simulink model "showKeyPoint"  (R2015a)
settings: Solver=ode45  StartTime=0.0  StopTime=10.0  RelTol=1e-3
InitFcn:
  | %% DSPBuilder Start
  | alt_dspbuilder_update_model(bdroot)
  | %% DSPBuilder End
libraries: allblocks_alteradspbuilder2 x340
(part 1 of 5)
settings Model: Creator=ASUS  LastModifiedBy=ASUS

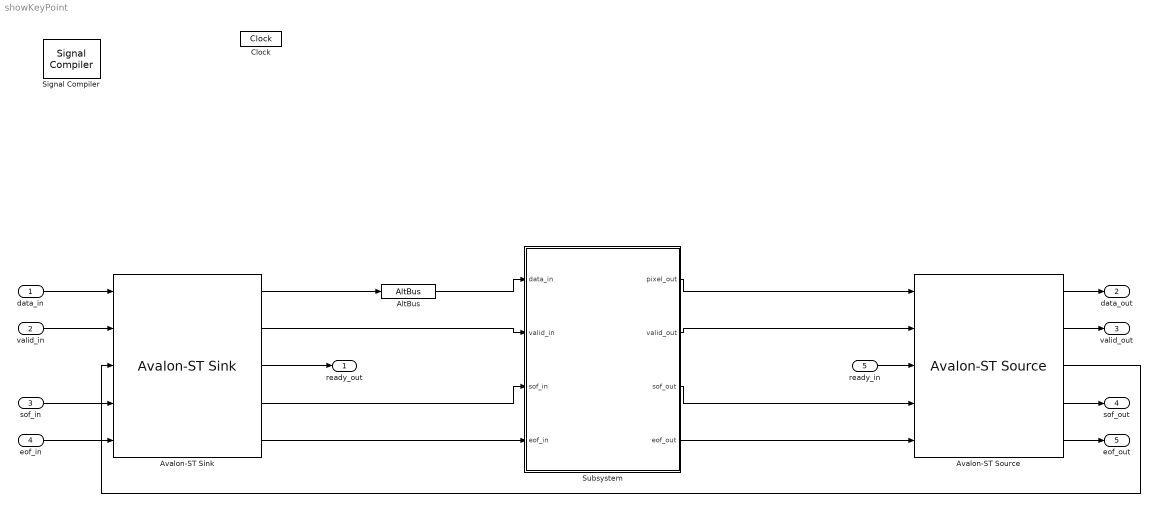
== system showKeyPoint ==
  data_in : Inport
  valid_in : Inport  Port=2
  sof_in : Inport  Port=3
  eof_in : Inport  Port=4
  ready_in : Inport  Port=5
  AltBus : allblocks_alteradspbuilder2/AltBus  BusType=Unsigned Integer  bwl=8  bwr=0  saturate=off  floatingPointInput=on  floatingPointOutput=on  logOutputs=off  logFile=C:\Users\ASUS\Desktop\sift_fpga_final\Gaussian filter 5x5\tb_gauss\gauss_AltBus.fixedpointlog
  Avalon-ST Sink : allblocks_alteradspbuilder2/Avalon-ST Sink  iofile=C:\Users\ASUS\Desktop\sift_fpga_final\Gaussian filter 5x5\tb_gauss\gauss_Avalon-ST+Sink_data.salt,C:\Users\ASUS\Desktop\sift_fpga_final\Gaussian filter 5x5\tb_gauss\gauss_Avalon-ST+Sink_valid.salt,C:\Users\ASUS\Desktop\sift_fpga_final\Gaussian filter 5x5\tb_gauss\gauss_Avalon-ST+Sink_ready.capture,C:\Users\ASUS\Desktop\sift_fpga_final\Gaussian filter 5x5\tb_gauss\gauss_Avalon-ST+Sink_startofpacket.salt,C:\Users\ASUS\Desktop\sift_fpga_final\Gaussian filter 5x5\tb_gauss\gauss_Avalon-ST+Sink_endofpacket.salt,  SpecifyClock=off  BusType=Unsigned Integer  bwl=24  bwr=0  symbolWidth=8  symbolsPerBeat=3  numOfChannels=0  numOfErrorDescriptors=0  endOfPacket=on  startOfPacket=on  empty=off  readyLatency=1  externalType=Inferred  PORTTYPE=Output
  Avalon-ST Source : allblocks_alteradspbuilder2/Avalon-ST Source  iofile=C:\Users\ASUS\Desktop\sift_fpga_final\Gaussian filter 5x5\tb_gauss\gauss_Avalon-ST+Source_data.capture,C:\Users\ASUS\Desktop\sift_fpga_final\Gaussian filter 5x5\tb_gauss\gauss_Avalon-ST+Source_valid.capture,C:\Users\ASUS\Desktop\sift_fpga_final\Gaussian filter 5x5\tb_gauss\gauss_Avalon-ST+Source_ready.salt,C:\Users\ASUS\Desktop\sift_fpga_final\Gaussian filter 5x5\tb_gauss\gauss_Avalon-ST+Source_startofpacket.capture,C:\Users\ASUS\Desktop\sift_fpga_final\Gaussian filter 5x5\tb_gauss\gauss_Avalon-ST+Source_endofpacket.capture,  SpecifyClock=off  BusType=Unsigned Integer  bwl=24  bwr=0  symbolWidth=8  symbolsPerBeat=3  numOfChannels=0  numOfErrorDescriptors=0  endOfPacket=on  startOfPacket=on  empty=off  readyLatency=1  externalType=Inferred  PORTTYPE=Input
  Clock : allblocks_alteradspbuilder2/Clock  ClockPeriod=20  ClockPeriodUnit=ns  SampleTime=1  ResetLatency=0  ResetRegisterCascadeDepth=0  SimulationStartCycle=5  PhaseOffset=0  Reset=aclr  ResetType=Active Low  Export=off
  Signal Compiler : allblocks_alteradspbuilder2/Signal Compiler  DeviceFamily=Stratix IV  DeviceName=AUTO  DisableEarlyHDLGeneration=off  EnableSignalTap=off  SignalTapDepth=128  UseBoardBlock=off  StpUseDefaultClock=on  StpClock=clock  ExportDir=.  MAX10_ProgrammingMode=Internal Flash (SDM) Single Boot
  Subsystem : Subsystem
  ready_out : Outport
  data_out : Outport  Port=2
  valid_out : Outport  Port=3
  sof_out : Outport  Port=4
  eof_out : Outport  Port=5
  wires:
  data_in/1 -> Avalon-ST Sink/1
  valid_in/1 -> Avalon-ST Sink/2
  sof_in/1 -> Avalon-ST Sink/4
  eof_in/1 -> Avalon-ST Sink/5
  ready_in/1 -> Avalon-ST Source/3
  Avalon-ST Sink/3 -> ready_out/1
  Avalon-ST Source/1 -> data_out/1
  Avalon-ST Source/2 -> valid_out/1
  Avalon-ST Source/4 -> sof_out/1
  Avalon-ST Source/5 -> eof_out/1
  Avalon-ST Sink/1 -> AltBus/1
  Subsystem/1(pixel_out) -> Avalon-ST Source/1
  Avalon-ST Sink/2 -> Subsystem/2(valid_in)
  Subsystem/2(valid_out) -> Avalon-ST Source/2
  Avalon-ST Sink/4 -> Subsystem/3(sof_in)
  Avalon-ST Sink/5 -> Subsystem/4(eof_in)
  Subsystem/3(sof_out) -> Avalon-ST Source/4
  Subsystem/4(eof_out) -> Avalon-ST Source/5
  Avalon-ST Source/3 -> Avalon-ST Sink/3
  AltBus/1 -> Subsystem/1(data_in)

== system showKeyPoint/Subsystem ==
  data_in : Inport
  valid_in : Inport  Port=2
  sof_in : Inport  Port=3
  eof_in : Inport  Port=4
  Bus Concatenation : allblocks_alteradspbuilder2/Bus Concatenation  isSigned=off  awidth=8  bwidth=8  pipeline_display=0
  Bus Concatenation1 : allblocks_alteradspbuilder2/Bus Concatenation  isSigned=off  awidth=8  bwidth=16  pipeline_display=0
  Memory Delay : allblocks_alteradspbuilder2/Memory Delay  BusType=Inferred  bwl=8  bwr=0  pipeline=4*640+28  pipeline_display=2588  ram_type=AUTO  use_ena=on  use_sclr=on  allowFloatingPointOverride=on  logOutputs=off  logFile=C:\Users\ASUS\Desktop\sift_fpga_final\Gaussian filter 5x5\tb_gauss\gauss_Subsystem_Memory+Delay.fixedpointlog
  Memory Delay1 : allblocks_alteradspbuilder2/Memory Delay  BusType=Inferred  bwl=8  bwr=0  pipeline=640*2+25  pipeline_display=1305  ram_type=AUTO  use_ena=on  use_sclr=on  allowFloatingPointOverride=on  logOutputs=off  logFile=C:\Users\ASUS\Desktop\sift_fpga_final\Gaussian filter 5x5\tb_gauss\gauss_Subsystem_Memory+Delay1.fixedpointlog
  Memory Delay2 : allblocks_alteradspbuilder2/Memory Delay  BusType=Inferred  bwl=8  bwr=0  pipeline=4*640+28  pipeline_display=2588  ram_type=AUTO  use_ena=on  use_sclr=on  allowFloatingPointOverride=on  logOutputs=off  logFile=C:\Users\ASUS\Desktop\sift_fpga_final\Gaussian filter 5x5\tb_gauss\gauss_Subsystem_Memory+Delay2.fixedpointlog
  find_keyPoint : Subsystem
  line_buff_3x3 : Subsystem
  pixel_out : Outport
  valid_out : Outport  Port=2
  sof_out : Outport  Port=3
  eof_out : Outport  Port=4
  wires:
  data_in/1 -> find_keyPoint/1(data_in), Memory Delay1/1
  Bus Concatenation/1 -> Bus Concatenation1/2
  find_keyPoint/1(is_keypoint) -> line_buff_3x3/2(is_keypoint)
  sof_in/1 -> Memory Delay/1, Memory Delay2/3, Memory Delay/3, line_buff_3x3/4(sclr), find_keyPoint/5(sclr), Memory Delay1/3, find_keyPoint/3(sof_in)
  valid_in/1 -> line_buff_3x3/3(clken), valid_out/1, Memory Delay/2, Memory Delay2/2, find_keyPoint/2(valid_in), Memory Delay1/2
  Memory Delay1/1 -> Bus Concatenation/1, Bus Concatenation1/1, Bus Concatenation/2
  line_buff_3x3/1(Out00) -> pixel_out/1
  Memory Delay/1 -> sof_out/1
  Bus Concatenation1/1 -> line_buff_3x3/1(dataIn)
  Memory Delay2/1 -> eof_out/1
  eof_in/1 -> Memory Delay2/1, find_keyPoint/4(eof_in)

== system showKeyPoint/Subsystem/find_keyPoint ==
  data_in : Inport
  valid_in : Inport  Port=2
  sof_in : Inport  Port=3
  eof_in : Inport  Port=4
  sclr : Inport  Port=5
  calculate_key_point : Subsystem
  dog_space : Subsystem
  scale_space : Subsystem
  is_keypoint : Outport
  wires:
  scale_space/3(scale2) -> dog_space/3(scale2_in)
  scale_space/1(scale4) -> dog_space/1(scale4_in)
  scale_space/2(scale3) -> dog_space/2(scale3_in)
  scale_space/4(scale1) -> dog_space/4(scale1_in)
  [pixel_in] -> scale_space/1(data_in)
  [valid_in] -> calculate_key_point/4(valid_in)
  dog_space/2(dog2_out) -> calculate_key_point/2(pixel_dog2_in)
  dog_space/1(dog3_out) -> calculate_key_point/1(pixel_dog3_in)
  valid_in/1 -> [valid_in]
  dog_space/3(dog1_out) -> calculate_key_point/3(pixel_dog1_in)
  data_in/1 -> [pixel_in]
  [valid_in] -> scale_space/2(valid_in)
  eof_in/1 -> [eof_in]
  sof_in/1 -> [sof_in]
  [valid_in] -> dog_space/5(valid_in)
  [sclr] -> dog_space/6(sclr)
  [sclr] -> calculate_key_point/5(sclr)
  [sclr] -> scale_space/3(sclr)
  calculate_key_point/1(is_KeyPoint) -> is_keypoint/1
  sclr/1 -> [sclr]

== system showKeyPoint/Subsystem/line_buff_3x3 ==
  dataIn : Inport
  is_keypoint : Inport  Port=2
  clken : Inport  Port=3
  sclr : Inport  Port=4
  Constant : allblocks_alteradspbuilder2/Constant  mask_cst=16711680  BusType=Unsigned Integer  bwl=24  bwr=0  roundMode=Truncate  satMode=Wrap  SpecifyClock=off  allowFloatingPointOverride=on  logOutputs=off  logFile=C:\Users\ASUS\Desktop\sift_fpga_final\Gaussian filter 5x5\tb_gauss\gauss_Subsystem_line%5Fbuff%5F3x3_Constant.fixedpointlog
  Constant1 : allblocks_alteradspbuilder2/Constant  mask_cst=16711680  BusType=Unsigned Integer  bwl=24  bwr=0  roundMode=Truncate  satMode=Wrap  SpecifyClock=off  allowFloatingPointOverride=on  logOutputs=off  logFile=C:\Users\ASUS\Desktop\sift_fpga_final\Gaussian filter 5x5\tb_gauss\gauss_Subsystem_line%5Fbuff%5F3x3_Constant1.fixedpointlog
  Constant2 : allblocks_alteradspbuilder2/Constant  mask_cst=16711680  BusType=Unsigned Integer  bwl=24  bwr=0  roundMode=Truncate  satMode=Wrap  SpecifyClock=off  allowFloatingPointOverride=on  logOutputs=off  logFile=C:\Users\ASUS\Desktop\sift_fpga_final\Gaussian filter 5x5\tb_gauss\gauss_Subsystem_line%5Fbuff%5F3x3_Constant2.fixedpointlog
  Constant3 : allblocks_alteradspbuilder2/Constant  mask_cst=16711680  BusType=Unsigned Integer  bwl=24  bwr=0  roundMode=Truncate  satMode=Wrap  SpecifyClock=off  allowFloatingPointOverride=on  logOutputs=off  logFile=C:\Users\ASUS\Desktop\sift_fpga_final\Gaussian filter 5x5\tb_gauss\gauss_Subsystem_line%5Fbuff%5F3x3_Constant3.fixedpointlog
  Constant4 : allblocks_alteradspbuilder2/Constant  mask_cst=16711680  BusType=Unsigned Integer  bwl=24  bwr=0  roundMode=Truncate  satMode=Wrap  SpecifyClock=off  allowFloatingPointOverride=on  logOutputs=off  logFile=C:\Users\ASUS\Desktop\sift_fpga_final\Gaussian filter 5x5\tb_gauss\gauss_Subsystem_line%5Fbuff%5F3x3_Constant4.fixedpointlog
  Constant5 : allblocks_alteradspbuilder2/Constant  mask_cst=16711680  BusType=Unsigned Integer  bwl=24  bwr=0  roundMode=Truncate  satMode=Wrap  SpecifyClock=off  allowFloatingPointOverride=on  logOutputs=off  logFile=C:\Users\ASUS\Desktop\sift_fpga_final\Gaussian filter 5x5\tb_gauss\gauss_Subsystem_line%5Fbuff%5F3x3_Constant5.fixedpointlog
  Constant6 : allblocks_alteradspbuilder2/Constant  mask_cst=16711680  BusType=Unsigned Integer  bwl=24  bwr=0  roundMode=Truncate  satMode=Wrap  SpecifyClock=off  allowFloatingPointOverride=on  logOutputs=off  logFile=C:\Users\ASUS\Desktop\sift_fpga_final\Gaussian filter 5x5\tb_gauss\gauss_Subsystem_line%5Fbuff%5F3x3_Constant6.fixedpointlog
  Constant7 : allblocks_alteradspbuilder2/Constant  mask_cst=16711680  BusType=Unsigned Integer  bwl=24  bwr=0  roundMode=Truncate  satMode=Wrap  SpecifyClock=off  allowFloatingPointOverride=on  logOutputs=off  logFile=C:\Users\ASUS\Desktop\sift_fpga_final\Gaussian filter 5x5\tb_gauss\gauss_Subsystem_line%5Fbuff%5F3x3_Constant7.fixedpointlog
  Constant8 : allblocks_alteradspbuilder2/Constant  mask_cst=16711680  BusType=Unsigned Integer  bwl=24  bwr=0  roundMode=Truncate  satMode=Wrap  SpecifyClock=off  allowFloatingPointOverride=on  logOutputs=off  logFile=C:\Users\ASUS\Desktop\sift_fpga_final\Gaussian filter 5x5\tb_gauss\gauss_Subsystem_line%5Fbuff%5F3x3_Constant8.fixedpointlog
  Delay : allblocks_alteradspbuilder2/Delay  pipeline=1  pipeline_display=1  ClockPhase=1  use_ena=on  use_sclr=on  allowFloatingPointOverride=on  logOutputs=off  logFile=C:\Users\ASUS\Desktop\sift_fpga_final\Gaussian filter 5x5\tb_gauss\gauss_Subsystem_line%5Fbuff%5F3x3_Delay.fixedpointlog  use_init=on  reset_value=0
  Delay1 : allblocks_alteradspbuilder2/Delay  pipeline=1  pipeline_display=1  ClockPhase=1  use_ena=on  use_sclr=on  allowFloatingPointOverride=on  logOutputs=off  logFile=C:\Users\ASUS\Desktop\sift_fpga_final\Gaussian filter 5x5\tb_gauss\gauss_Subsystem_line%5Fbuff%5F3x3_Delay1.fixedpointlog  use_init=on  reset_value=0
  Delay10 : allblocks_alteradspbuilder2/Delay  pipeline=1  pipeline_display=1  ClockPhase=1  use_ena=on  use_sclr=on  allowFloatingPointOverride=on  logOutputs=off  logFile=C:\Users\ASUS\Desktop\sift_fpga_final\Gaussian filter 5x5\tb_gauss\gauss_Subsystem_line%5Fbuff%5F3x3_Delay10.fixedpointlog  use_init=on  reset_value=0
  Delay2 : allblocks_alteradspbuilder2/Delay  pipeline=1  pipeline_display=1  ClockPhase=1  use_ena=on  use_sclr=on  allowFloatingPointOverride=on  logOutputs=off  logFile=C:\Users\ASUS\Desktop\sift_fpga_final\Gaussian filter 5x5\tb_gauss\gauss_Subsystem_line%5Fbuff%5F3x3_Delay2.fixedpointlog  use_init=on  reset_value=0
  Delay5 : allblocks_alteradspbuilder2/Delay  pipeline=1  pipeline_display=1  ClockPhase=1  use_ena=on  use_sclr=on  allowFloatingPointOverride=on  logOutputs=off  logFile=C:\Users\ASUS\Desktop\sift_fpga_final\Gaussian filter 5x5\tb_gauss\gauss_Subsystem_line%5Fbuff%5F3x3_Delay5.fixedpointlog  use_init=on  reset_value=0
  Delay6 : allblocks_alteradspbuilder2/Delay  pipeline=1  pipeline_display=1  ClockPhase=1  use_ena=on  use_sclr=on  allowFloatingPointOverride=on  logOutputs=off  logFile=C:\Users\ASUS\Desktop\sift_fpga_final\Gaussian filter 5x5\tb_gauss\gauss_Subsystem_line%5Fbuff%5F3x3_Delay6.fixedpointlog  use_init=on  reset_value=0
  Delay9 : allblocks_alteradspbuilder2/Delay  pipeline=1  pipeline_display=1  ClockPhase=1  use_ena=on  use_sclr=on  allowFloatingPointOverride=on  logOutputs=off  logFile=C:\Users\ASUS\Desktop\sift_fpga_final\Gaussian filter 5x5\tb_gauss\gauss_Subsystem_line%5Fbuff%5F3x3_Delay9.fixedpointlog  use_init=on  reset_value=0
  Memory Delay : allblocks_alteradspbuilder2/Memory Delay  BusType=Unsigned Integer  bwl=8  bwr=0  pipeline=638  pipeline_display=638  ram_type=AUTO  use_ena=on  use_sclr=on  allowFloatingPointOverride=on  logOutputs=off  logFile=C:\Users\ASUS\Desktop\sift_fpga_final\Gaussian filter 5x5\tb_gauss\gauss_Subsystem_line%5Fbuff%5F3x3_Memory+Delay.fixedpointlog
  Memory Delay1 : allblocks_alteradspbuilder2/Memory Delay  BusType=Unsigned Integer  bwl=8  bwr=0  pipeline=638  pipeline_display=638  ram_type=AUTO  use_ena=on  use_sclr=on  allowFloatingPointOverride=on  logOutputs=off  logFile=C:\Users\ASUS\Desktop\sift_fpga_final\Gaussian filter 5x5\tb_gauss\gauss_Subsystem_line%5Fbuff%5F3x3_Memory+Delay1.fixedpointlog
  Multiplexer : allblocks_alteradspbuilder2/Multiplexer  numInputs=2  pipeline=0  oneHot=off  pipeline_display=0  use_ena=off  use_aclr=off  allowFloatingPointOverride=on  logOutputs=off  logFile=C:\Users\ASUS\Desktop\sift_fpga_final\Gaussian filter 5x5\tb_gauss\gauss_Subsystem_line%5Fbuff%5F3x3_Multiplexer.fixedpointlog
  Multiplexer1 : allblocks_alteradspbuilder2/Multiplexer  numInputs=2  pipeline=0  oneHot=off  pipeline_display=0  use_ena=off  use_aclr=off  allowFloatingPointOverride=on  logOutputs=off  logFile=C:\Users\ASUS\Desktop\sift_fpga_final\Gaussian filter 5x5\tb_gauss\gauss_Subsystem_line%5Fbuff%5F3x3_Multiplexer1.fixedpointlog
  Multiplexer2 : allblocks_alteradspbuilder2/Multiplexer  numInputs=2  pipeline=0  oneHot=off  pipeline_display=0  use_ena=off  use_aclr=off  allowFloatingPointOverride=on  logOutputs=off  logFile=C:\Users\ASUS\Desktop\sift_fpga_final\Gaussian filter 5x5\tb_gauss\gauss_Subsystem_line%5Fbuff%5F3x3_Multiplexer2.fixedpointlog
  Multiplexer3 : allblocks_alteradspbuilder2/Multiplexer  numInputs=2  pipeline=0  oneHot=off  pipeline_display=0  use_ena=off  use_aclr=off  allowFloatingPointOverride=on  logOutputs=off  logFile=C:\Users\ASUS\Desktop\sift_fpga_final\Gaussian filter 5x5\tb_gauss\gauss_Subsystem_line%5Fbuff%5F3x3_Multiplexer3.fixedpointlog
  Multiplexer4 : allblocks_alteradspbuilder2/Multiplexer  numInputs=2  pipeline=0  oneHot=off  pipeline_display=0  use_ena=off  use_aclr=off  allowFloatingPointOverride=on  logOutputs=off  logFile=C:\Users\ASUS\Desktop\sift_fpga_final\Gaussian filter 5x5\tb_gauss\gauss_Subsystem_line%5Fbuff%5F3x3_Multiplexer4.fixedpointlog
  Multiplexer5 : allblocks_alteradspbuilder2/Multiplexer  numInputs=2  pipeline=0  oneHot=off  pipeline_display=0  use_ena=off  use_aclr=off  allowFloatingPointOverride=on  logOutputs=off  logFile=C:\Users\ASUS\Desktop\sift_fpga_final\Gaussian filter 5x5\tb_gauss\gauss_Subsystem_line%5Fbuff%5F3x3_Multiplexer5.fixedpointlog
  Multiplexer6 : allblocks_alteradspbuilder2/Multiplexer  numInputs=2  pipeline=0  oneHot=off  pipeline_display=0  use_ena=off  use_aclr=off  allowFloatingPointOverride=on  logOutputs=off  logFile=C:\Users\ASUS\Desktop\sift_fpga_final\Gaussian filter 5x5\tb_gauss\gauss_Subsystem_line%5Fbuff%5F3x3_Multiplexer6.fixedpointlog
  Multiplexer7 : allblocks_alteradspbuilder2/Multiplexer  numInputs=2  pipeline=0  oneHot=off  pipeline_display=0  use_ena=off  use_aclr=off  allowFloatingPointOverride=on  logOutputs=off  logFile=C:\Users\ASUS\Desktop\sift_fpga_final\Gaussian filter 5x5\tb_gauss\gauss_Subsystem_line%5Fbuff%5F3x3_Multiplexer7.fixedpointlog
  Multiplexer8 : allblocks_alteradspbuilder2/Multiplexer  numInputs=2  pipeline=0  oneHot=off  pipeline_display=0  use_ena=off  use_aclr=off  allowFloatingPointOverride=on  logOutputs=off  logFile=C:\Users\ASUS\Desktop\sift_fpga_final\Gaussian filter 5x5\tb_gauss\gauss_Subsystem_line%5Fbuff%5F3x3_Multiplexer8.fixedpointlog
  Out00 : Outport
  wires:
  [clken] -> Delay10/2
  [clken] -> Memory Delay1/2
  [clken] -> Delay9/2
  [clken] -> Delay1/2
  [clken] -> Delay/2
  [data_in] -> Delay/1
  [clken] -> Delay2/2
  Multiplexer8/1 -> Memory Delay/1
  clken/1 -> [clken]
  [clken] -> Memory Delay/2
  [clken] -> Delay6/2
  [pixel_out] -> Out00/1
  [clken] -> Delay5/2
  dataIn/1 -> [data_in]
  sclr/1 -> [sclr]
  [sclr] -> Delay/3
  [sclr] -> Delay1/3
  [sclr] -> Delay2/3
  [sclr] -> Memory Delay/3
  [sclr] -> Delay5/3
  [sclr] -> Delay6/3
  [sclr] -> Memory Delay1/3
  [sclr] -> Delay9/3
  [sclr] -> Delay10/3
  [is_keypoint] -> Multiplexer/1
  is_keypoint/1 -> [is_keypoint]
  Multiplexer/1 -> Delay1/1
  Delay/1 -> Multiplexer/2
  [is_keypoint] -> Multiplexer1/1
  Multiplexer1/1 -> Delay2/1
  Delay1/1 -> Multiplexer1/2
  Constant1/1 -> Multiplexer1/3
  [is_keypoint] -> Multiplexer2/1
  Multiplexer2/1 -> Delay5/1
  Memory Delay/1 -> Multiplexer2/2
  Constant2/1 -> Multiplexer2/3
  [is_keypoint] -> Multiplexer3/1
  Multiplexer3/1 -> Delay6/1
  Delay5/1 -> Multiplexer3/2
  Constant3/1 -> Multiplexer3/3
  [is_keypoint] -> Multiplexer4/1
  Multiplexer4/1 -> Memory Delay1/1
  Delay6/1 -> Multiplexer4/2
  Constant4/1 -> Multiplexer4/3
  [is_keypoint] -> Multiplexer5/1
  Multiplexer5/1 -> Delay9/1
  Memory Delay1/1 -> Multiplexer5/2
  Constant5/1 -> Multiplexer5/3
  [is_keypoint] -> Multiplexer6/1
  Multiplexer6/1 -> Delay10/1
  Delay9/1 -> Multiplexer6/2
  Constant6/1 -> Multiplexer6/3
  [is_keypoint] -> Multiplexer7/1
  Multiplexer7/1 -> [pixel_out]
  Delay10/1 -> Multiplexer7/2
  Constant7/1 -> Multiplexer7/3
  Constant/1 -> Multiplexer/3
  [is_keypoint] -> Multiplexer8/1
  Delay2/1 -> Multiplexer8/2
  Constant8/1 -> Multiplexer8/3

== system showKeyPoint/Subsystem/find_keyPoint/calculate_key_point ==
  pixel_dog3_in : Inport
  pixel_dog2_in : Inport  Port=2
  pixel_dog1_in : Inport  Port=3
  valid_in : Inport  Port=4
  sclr : Inport  Port=5
  find_KeyPoint : Subsystem
  line_buff_3x1 : Subsystem
  line_buff_3x2 : Subsystem
  line_buff_3x3 : Subsystem
  is_KeyPoint : Outport
  wires:
  line_buff_3x3/3(Out02) -> find_KeyPoint/3(dataIn_12)
  line_buff_3x3/6(Out12) -> find_KeyPoint/6(dataIn_15)
  line_buff_3x3/4(Out10) -> find_KeyPoint/4(dataIn_13)
  line_buff_3x3/5(Out11) -> find_KeyPoint/5(dataIn_14)
  line_buff_3x1/2(Out01) -> find_KeyPoint/11(dataIn_21)
  line_buff_3x1/3(Out02) -> find_KeyPoint/12(dataIn_22)
  line_buff_3x1/4(Out10) -> find_KeyPoint/13(dataIn_23)
  line_buff_3x3/2(Out01) -> find_KeyPoint/2(dataIn_11)
  line_buff_3x2/8(Out21) -> find_KeyPoint/26(dataIn_37)
  line_buff_3x3/8(Out21) -> find_KeyPoint/8(dataIn_17)
  line_buff_3x3/1(Out00) -> find_KeyPoint/1(dataIn_10)
  line_buff_3x3/7(Out20) -> find_KeyPoint/7(dataIn_16)
  line_buff_3x3/9(Out22) -> find_KeyPoint/9(dataIn_18)
  line_buff_3x1/1(Out00) -> find_KeyPoint/10(dataIn_20)
  line_buff_3x2/7(Out20) -> find_KeyPoint/25(dataIn_36)
  [pixel_dog2_in] -> line_buff_3x1/1(dataIn)
  [pixel_dog1_in] -> line_buff_3x3/1(dataIn)
  [valid_in] -> line_buff_3x2/2(clken)
  valid_in/1 -> [valid_in]
  [valid_in] -> line_buff_3x1/2(clken)
  pixel_dog2_in/1 -> [pixel_dog2_in]
  pixel_dog1_in/1 -> [pixel_dog1_in]
  pixel_dog3_in/1 -> [pixel_dog3_in]
  [valid_in] -> line_buff_3x3/2(clken)
  [pixel_dog3_in] -> line_buff_3x2/1(dataIn)
  line_buff_3x2/2(Out01) -> find_KeyPoint/20(dataIn_31)
  line_buff_3x2/3(Out02) -> find_KeyPoint/21(dataIn_32)
  line_buff_3x2/4(Out10) -> find_KeyPoint/22(dataIn_33)
  line_buff_3x2/5(Out11) -> find_KeyPoint/23(dataIn_34)
  line_buff_3x2/1(Out00) -> find_KeyPoint/19(dataIn_30)
  line_buff_3x1/5(Out11) -> find_KeyPoint/14(dataIn_24)
  line_buff_3x1/6(Out12) -> find_KeyPoint/15(dataIn_25)
  line_buff_3x1/7(Out20) -> find_KeyPoint/16(dataIn_26)
  line_buff_3x1/8(Out21) -> find_KeyPoint/17(dataIn_27)
  line_buff_3x2/6(Out12) -> find_KeyPoint/24(dataIn_35)
  line_buff_3x2/9(Out22) -> find_KeyPoint/27(dataIn_38)
  line_buff_3x1/9(Out22) -> find_KeyPoint/18(dataIn_28)
  find_KeyPoint/1(is_KeyPoint) -> is_KeyPoint/1
  sclr/1 -> [sclr]
  [sclr] -> line_buff_3x3/3(sclr)
  [sclr] -> line_buff_3x1/3(sclr)
  [sclr] -> line_buff_3x2/3(sclr)

== system showKeyPoint/Subsystem/find_keyPoint/dog_space ==
  scale4_in : Inport
  scale3_in : Inport  Port=2
  scale2_in : Inport  Port=3
  scale1_in : Inport  Port=4
  valid_in : Inport  Port=5
  sclr : Inport  Port=6
  Parallel Adder Subtractor : allblocks_alteradspbuilder2/Parallel Adder Subtractor  number_of_inputs=2  direction=+-  use_pipeline=on  pipeline_display=1  phase_selection=1  use_ena=on  use_aclr=on  allowFloatingPointOverride=on  logOutputs=off  logFile=C:\Users\ASUS\Desktop\sift_fpga_final\Gaussian filter 5x5\tb_gauss\gauss_Subsystem_find%5FkeyPoint_dog%5Fspace_Parallel+Adder+Subtractor.fixedpointlog
  Parallel Adder Subtractor1 : allblocks_alteradspbuilder2/Parallel Adder Subtractor  number_of_inputs=2  direction=+-  use_pipeline=on  pipeline_display=1  phase_selection=1  use_ena=on  use_aclr=on  allowFloatingPointOverride=on  logOutputs=off  logFile=C:\Users\ASUS\Desktop\sift_fpga_final\Gaussian filter 5x5\tb_gauss\gauss_Subsystem_find%5FkeyPoint_dog%5Fspace_Parallel+Adder+Subtractor1.fixedpointlog
  Parallel Adder Subtractor2 : allblocks_alteradspbuilder2/Parallel Adder Subtractor  number_of_inputs=2  direction=+-  use_pipeline=on  pipeline_display=1  phase_selection=1  use_ena=on  use_aclr=on  allowFloatingPointOverride=on  logOutputs=off  logFile=C:\Users\ASUS\Desktop\sift_fpga_final\Gaussian filter 5x5\tb_gauss\gauss_Subsystem_find%5FkeyPoint_dog%5Fspace_Parallel+Adder+Subtractor2.fixedpointlog
  dog3_out : Outport
  dog2_out : Outport  Port=2
  dog1_out : Outport  Port=3
  wires:
  [pixel_scale2] -> Parallel Adder Subtractor1/1
  Parallel Adder Subtractor1/1 -> dog1_out/1
  [pixel_scale3] -> Parallel Adder Subtractor/1
  [valid_in] -> Parallel Adder Subtractor2/3
  [pixel_scale2] -> Parallel Adder Subtractor/2
  [pixel_scale3] -> Parallel Adder Subtractor2/2
  Parallel Adder Subtractor/1 -> dog2_out/1
  [valid_in] -> Parallel Adder Subtractor1/3
  Parallel Adder Subtractor2/1 -> dog3_out/1
  [pixel_scale1] -> Parallel Adder Subtractor1/2
  [valid_in] -> Parallel Adder Subtractor/3
  [pixel_scale4] -> Parallel Adder Subtractor2/1
  scale4_in/1 -> [pixel_scale4]
  scale3_in/1 -> [pixel_scale3]
  scale2_in/1 -> [pixel_scale2]
  scale1_in/1 -> [pixel_scale1]
  valid_in/1 -> [valid_in]
  sclr/1 -> [sclr]
  [sclr] -> Parallel Adder Subtractor2/4
  [sclr] -> Parallel Adder Subtractor/4
  [sclr] -> Parallel Adder Subtractor1/4

== system showKeyPoint/Subsystem/find_keyPoint/scale_space ==
  data_in : Inport
  valid_in : Inport  Port=2
  sclr : Inport  Port=3
  Gaussian_scale1 : Subsystem
  Gaussian_scale2 : Subsystem
  Gaussian_scale3 : Subsystem
  Gaussian_scale4 : Subsystem
  scale4 : Outport
  scale3 : Outport  Port=2
  scale2 : Outport  Port=3
  scale1 : Outport  Port=4
  wires:
  data_in/1 -> [pixel_in]
  valid_in/1 -> [valid_in]
  [pixel_in] -> Gaussian_scale3/1(pixel_in)
  [pixel_in] -> Gaussian_scale4/1(pixel_in)
  [valid_in] -> Gaussian_scale3/2(valid_in)
  [pixel_in] -> Gaussian_scale1/1(pixel_in)
  [valid_in] -> Gaussian_scale1/2(valid_in)
  [valid_in] -> Gaussian_scale4/2(valid_in)
  [pixel_in] -> Gaussian_scale2/1(pixel_in)
  [valid_in] -> Gaussian_scale2/2(valid_in)
  Gaussian_scale3/1(pixel_out) -> [pixel_scale3]
  [pixel_scale3] -> scale3/1
  [pixel_scale2] -> scale2/1
  Gaussian_scale4/1(pixel_out) -> [pixel_scale4]
  [pixel_scale4] -> scale4/1
  Gaussian_scale1/1(pixel_out) -> [pixel_scale1]
  Gaussian_scale2/1(pixel_out) -> [pixel_scale2]
  [pixel_scale1] -> scale1/1
  sclr/1 -> [sclr]
  [sclr] -> Gaussian_scale4/3(sclr)
  [sclr] -> Gaussian_scale3/3(sclr)
  [sclr] -> Gaussian_scale2/3(sclr)
  [sclr] -> Gaussian_scale1/3(sclr)

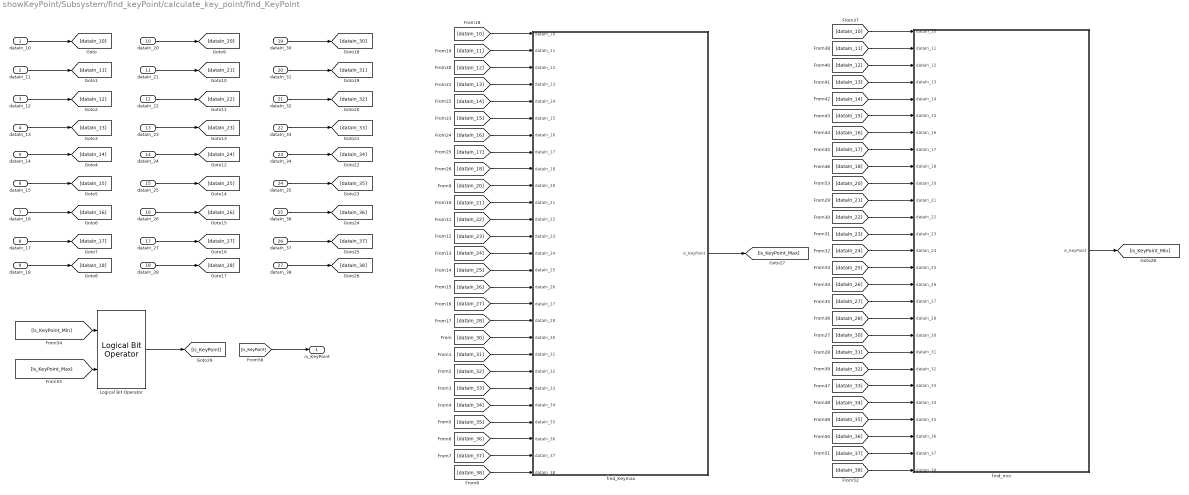
== system showKeyPoint/Subsystem/find_keyPoint/calculate_key_point/find_KeyPoint ==
  dataIn_10 : Inport
  dataIn_11 : Inport  Port=2
  dataIn_12 : Inport  Port=3
  dataIn_13 : Inport  Port=4
  dataIn_14 : Inport  Port=5
  dataIn_15 : Inport  Port=6
  dataIn_16 : Inport  Port=7
  dataIn_17 : Inport  Port=8
  dataIn_18 : Inport  Port=9
  dataIn_20 : Inport  Port=10
  dataIn_21 : Inport  Port=11
  dataIn_22 : Inport  Port=12
  dataIn_23 : Inport  Port=13
  dataIn_24 : Inport  Port=14
  dataIn_25 : Inport  Port=15
  dataIn_26 : Inport  Port=16
  dataIn_27 : Inport  Port=17
  dataIn_28 : Inport  Port=18
  dataIn_30 : Inport  Port=19
  dataIn_31 : Inport  Port=20
  dataIn_32 : Inport  Port=21
  dataIn_33 : Inport  Port=22
  dataIn_34 : Inport  Port=23
  dataIn_35 : Inport  Port=24
  dataIn_36 : Inport  Port=25
  dataIn_37 : Inport  Port=26
  dataIn_38 : Inport  Port=27
  Logical Bit Operator : allblocks_alteradspbuilder2/Logical Bit Operator  LogicalOperator=OR  user_inputs=2  pipeline_display=0
  find_Keymax : Subsystem
  find_min : Subsystem
  is_KeyPoint : Outport
  wires:
  [dataIn_32] -> find_Keymax/21(dataIn_32)
  [dataIn_33] -> find_Keymax/22(dataIn_33)
  [dataIn_36] -> find_Keymax/25(dataIn_36)
  [dataIn_37] -> find_Keymax/26(dataIn_37)
  [dataIn_34] -> find_Keymax/23(dataIn_34)
  [dataIn_35] -> find_Keymax/24(dataIn_35)
  [dataIn_30] -> find_Keymax/19(dataIn_30)
  [dataIn_31] -> find_Keymax/20(dataIn_31)
  [is_KeyPoint_Max] -> Logical Bit Operator/2
  [is_KeyPoint_Min] -> Logical Bit Operator/1
  find_Keymax/1(is_KeyPoint) -> [is_KeyPoint_Max]
  [dataIn_28] -> find_Keymax/18(dataIn_28)
  [dataIn_26] -> find_Keymax/16(dataIn_26)
  [dataIn_22] -> find_Keymax/12(dataIn_22)
  [dataIn_27] -> find_Keymax/17(dataIn_27)
  [dataIn_20] -> find_Keymax/10(dataIn_20)
  [dataIn_23] -> find_Keymax/13(dataIn_23)
  [dataIn_24] -> find_Keymax/14(dataIn_24)
  [dataIn_21] -> find_Keymax/11(dataIn_21)
  [dataIn_25] -> find_Keymax/15(dataIn_25)
  [dataIn_10] -> find_Keymax/1(dataIn_10)
  [dataIn_11] -> find_Keymax/2(dataIn_11)
  [dataIn_12] -> find_Keymax/3(dataIn_12)
  dataIn_23/1 -> [dataIn_23]
  dataIn_17/1 -> [dataIn_17]
  dataIn_22/1 -> [dataIn_22]
  dataIn_14/1 -> [dataIn_14]
  dataIn_16/1 -> [dataIn_16]
  dataIn_28/1 -> [dataIn_28]
  dataIn_20/1 -> [dataIn_20]
  dataIn_21/1 -> [dataIn_21]
  dataIn_26/1 -> [dataIn_26]
  dataIn_10/1 -> [dataIn_10]
  dataIn_30/1 -> [dataIn_30]
  dataIn_27/1 -> [dataIn_27]
  dataIn_25/1 -> [dataIn_25]
  dataIn_15/1 -> [dataIn_15]
  dataIn_18/1 -> [dataIn_18]
  dataIn_24/1 -> [dataIn_24]
  dataIn_32/1 -> [dataIn_32]
  dataIn_13/1 -> [dataIn_13]
  dataIn_31/1 -> [dataIn_31]
  [dataIn_14] -> find_Keymax/5(dataIn_14)
  dataIn_34/1 -> [dataIn_34]
  dataIn_11/1 -> [dataIn_11]
  [dataIn_17] -> find_Keymax/8(dataIn_17)
  dataIn_35/1 -> [dataIn_35]
  dataIn_33/1 -> [dataIn_33]
  dataIn_38/1 -> [dataIn_38]
  [dataIn_13] -> find_Keymax/4(dataIn_13)
  [dataIn_16] -> find_Keymax/7(dataIn_16)
  [dataIn_15] -> find_Keymax/6(dataIn_15)
  dataIn_12/1 -> [dataIn_12]
  [dataIn_18] -> find_Keymax/9(dataIn_18)
  dataIn_36/1 -> [dataIn_36]
  dataIn_37/1 -> [dataIn_37]
  [dataIn_38] -> find_Keymax/27(dataIn_38)
  find_min/1(is_KeyPoint) -> [is_KeyPoint_Min]
  [dataIn_11] -> find_min/2(dataIn_11)
  [dataIn_12] -> find_min/3(dataIn_12)
  [dataIn_13] -> find_min/4(dataIn_13)
  [dataIn_15] -> find_min/6(dataIn_15)
  [dataIn_16] -> find_min/7(dataIn_16)
  [dataIn_17] -> find_min/8(dataIn_17)
  [dataIn_18] -> find_min/9(dataIn_18)
  [dataIn_31] -> find_min/20(dataIn_31)
  [dataIn_14] -> find_min/5(dataIn_14)
  [is_KeyPoint] -> is_KeyPoint/1
  [dataIn_33] -> find_min/22(dataIn_33)
  [dataIn_32] -> find_min/21(dataIn_32)
  [dataIn_34] -> find_min/23(dataIn_34)
  [dataIn_35] -> find_min/24(dataIn_35)
  [dataIn_36] -> find_min/25(dataIn_36)
  [dataIn_21] -> find_min/11(dataIn_21)
  [dataIn_22] -> find_min/12(dataIn_22)
  [dataIn_23] -> find_min/13(dataIn_23)
  [dataIn_25] -> find_min/15(dataIn_25)
  [dataIn_24] -> find_min/14(dataIn_24)
  [dataIn_38] -> find_min/27(dataIn_38)
  [dataIn_20] -> find_min/10(dataIn_20)
  [dataIn_26] -> find_min/16(dataIn_26)
  [dataIn_30] -> find_min/19(dataIn_30)
  [dataIn_27] -> find_min/17(dataIn_27)
  [dataIn_37] -> find_min/26(dataIn_37)
  [dataIn_28] -> find_min/18(dataIn_28)
  [dataIn_10] -> find_min/1(dataIn_10)
  Logical Bit Operator/1 -> [is_KeyPoint]

== system showKeyPoint/Subsystem/find_keyPoint/calculate_key_point/line_buff_3x1 ==
  dataIn : Inport
  clken : Inport  Port=2
  sclr : Inport  Port=3
  Delay : allblocks_alteradspbuilder2/Delay  pipeline=1  pipeline_display=1  ClockPhase=1  use_ena=on  use_sclr=on  allowFloatingPointOverride=on  logOutputs=off  logFile=C:\Users\ASUS\Desktop\sift_fpga_final\Gaussian filter 5x5\tb_gauss\gauss_Subsystem_find%5FkeyPoint_calculate%5Fkey%5Fpoint_line%5Fbuff%5F3x1_Delay.fixedpointlog  use_init=on  reset_value=0
  Delay1 : allblocks_alteradspbuilder2/Delay  pipeline=1  pipeline_display=1  ClockPhase=1  use_ena=on  use_sclr=on  allowFloatingPointOverride=on  logOutputs=off  logFile=C:\Users\ASUS\Desktop\sift_fpga_final\Gaussian filter 5x5\tb_gauss\gauss_Subsystem_find%5FkeyPoint_calculate%5Fkey%5Fpoint_line%5Fbuff%5F3x1_Delay1.fixedpointlog  use_init=on  reset_value=0
  Delay10 : allblocks_alteradspbuilder2/Delay  pipeline=1  pipeline_display=1  ClockPhase=1  use_ena=on  use_sclr=on  allowFloatingPointOverride=on  logOutputs=off  logFile=C:\Users\ASUS\Desktop\sift_fpga_final\Gaussian filter 5x5\tb_gauss\gauss_Subsystem_find%5FkeyPoint_calculate%5Fkey%5Fpoint_line%5Fbuff%5F3x1_Delay10.fixedpointlog  use_init=on  reset_value=0
  Delay2 : allblocks_alteradspbuilder2/Delay  pipeline=1  pipeline_display=1  ClockPhase=1  use_ena=on  use_sclr=on  allowFloatingPointOverride=on  logOutputs=off  logFile=C:\Users\ASUS\Desktop\sift_fpga_final\Gaussian filter 5x5\tb_gauss\gauss_Subsystem_find%5FkeyPoint_calculate%5Fkey%5Fpoint_line%5Fbuff%5F3x1_Delay2.fixedpointlog  use_init=on  reset_value=0
  Delay5 : allblocks_alteradspbuilder2/Delay  pipeline=1  pipeline_display=1  ClockPhase=1  use_ena=on  use_sclr=on  allowFloatingPointOverride=on  logOutputs=off  logFile=C:\Users\ASUS\Desktop\sift_fpga_final\Gaussian filter 5x5\tb_gauss\gauss_Subsystem_find%5FkeyPoint_calculate%5Fkey%5Fpoint_line%5Fbuff%5F3x1_Delay5.fixedpointlog  use_init=on  reset_value=0
  Delay6 : allblocks_alteradspbuilder2/Delay  pipeline=1  pipeline_display=1  ClockPhase=1  use_ena=on  use_sclr=on  allowFloatingPointOverride=on  logOutputs=off  logFile=C:\Users\ASUS\Desktop\sift_fpga_final\Gaussian filter 5x5\tb_gauss\gauss_Subsystem_find%5FkeyPoint_calculate%5Fkey%5Fpoint_line%5Fbuff%5F3x1_Delay6.fixedpointlog  use_init=on  reset_value=0
  Delay9 : allblocks_alteradspbuilder2/Delay  pipeline=1  pipeline_display=1  ClockPhase=1  use_ena=on  use_sclr=on  allowFloatingPointOverride=on  logOutputs=off  logFile=C:\Users\ASUS\Desktop\sift_fpga_final\Gaussian filter 5x5\tb_gauss\gauss_Subsystem_find%5FkeyPoint_calculate%5Fkey%5Fpoint_line%5Fbuff%5F3x1_Delay9.fixedpointlog  use_init=on  reset_value=0
  Memory Delay : allblocks_alteradspbuilder2/Memory Delay  BusType=Unsigned Integer  bwl=8  bwr=0  pipeline=638  pipeline_display=638  ram_type=AUTO  use_ena=on  use_sclr=on  allowFloatingPointOverride=on  logOutputs=off  logFile=C:\Users\ASUS\Desktop\sift_fpga_final\Gaussian filter 5x5\tb_gauss\gauss_Subsystem_find%5FkeyPoint_calculate%5Fkey%5Fpoint_line%5Fbuff%5F3x1_Memory+Delay.fixedpointlog
  Memory Delay1 : allblocks_alteradspbuilder2/Memory Delay  BusType=Unsigned Integer  bwl=8  bwr=0  pipeline=638  pipeline_display=638  ram_type=AUTO  use_ena=on  use_sclr=on  allowFloatingPointOverride=on  logOutputs=off  logFile=C:\Users\ASUS\Desktop\sift_fpga_final\Gaussian filter 5x5\tb_gauss\gauss_Subsystem_find%5FkeyPoint_calculate%5Fkey%5Fpoint_line%5Fbuff%5F3x1_Memory+Delay1.fixedpointlog
  Out00 : Outport
  Out01 : Outport  Port=2
  Out02 : Outport  Port=3
  Out10 : Outport  Port=4
  Out11 : Outport  Port=5
  Out12 : Outport  Port=6
  Out20 : Outport  Port=7
  Out21 : Outport  Port=8
  Out22 : Outport  Port=9
  wires:
  Delay1/1 -> [data_01], Delay2/1
  Delay/1 -> [data_00], Delay1/1
  Delay9/1 -> [data_21], Delay10/1
  [clken] -> Delay10/2
  [clken] -> Memory Delay1/2
  Delay6/1 -> Memory Delay1/1, [data_12]
  Memory Delay1/1 -> [data_20], Delay9/1
  [clken] -> Delay9/2
  [data_02] -> Out02/1
  [clken] -> Delay1/2
  [clken] -> Delay/2
  [data_in] -> Delay/1
  [clken] -> Delay2/2
  Delay2/1 -> [data_02], Memory Delay/1
  [data_22] -> Out22/1
  Delay10/1 -> [data_22]
  clken/1 -> [clken]
  [data_21] -> Out21/1
  [data_20] -> Out20/1
  [data_10] -> Out10/1
  Memory Delay/1 -> [data_10], Delay5/1
  [clken] -> Memory Delay/2
  [clken] -> Delay6/2
  Delay5/1 -> [data_11], Delay6/1
  [data_12] -> Out12/1
  [data_00] -> Out00/1
  [data_01] -> Out01/1
  [clken] -> Delay5/2
  [data_11] -> Out11/1
  dataIn/1 -> [data_in]
  sclr/1 -> [sclr]
  [sclr] -> Delay/3
  [sclr] -> Delay1/3
  [sclr] -> Delay2/3
  [sclr] -> Memory Delay/3
  [sclr] -> Delay5/3
  [sclr] -> Delay6/3
  [sclr] -> Memory Delay1/3
  [sclr] -> Delay9/3
  [sclr] -> Delay10/3

== system showKeyPoint/Subsystem/find_keyPoint/calculate_key_point/line_buff_3x2 ==
  dataIn : Inport
  clken : Inport  Port=2
  sclr : Inport  Port=3
  Delay : allblocks_alteradspbuilder2/Delay  pipeline=1  pipeline_display=1  ClockPhase=1  use_ena=on  use_sclr=on  allowFloatingPointOverride=on  logOutputs=off  logFile=C:\Users\ASUS\Desktop\sift_fpga_final\Gaussian filter 5x5\tb_gauss\gauss_Subsystem_find%5FkeyPoint_calculate%5Fkey%5Fpoint_line%5Fbuff%5F3x2_Delay.fixedpointlog  use_init=on  reset_value=0
  Delay1 : allblocks_alteradspbuilder2/Delay  pipeline=1  pipeline_display=1  ClockPhase=1  use_ena=on  use_sclr=on  allowFloatingPointOverride=on  logOutputs=off  logFile=C:\Users\ASUS\Desktop\sift_fpga_final\Gaussian filter 5x5\tb_gauss\gauss_Subsystem_find%5FkeyPoint_calculate%5Fkey%5Fpoint_line%5Fbuff%5F3x2_Delay1.fixedpointlog  use_init=on  reset_value=0
  Delay10 : allblocks_alteradspbuilder2/Delay  pipeline=1  pipeline_display=1  ClockPhase=1  use_ena=on  use_sclr=on  allowFloatingPointOverride=on  logOutputs=off  logFile=C:\Users\ASUS\Desktop\sift_fpga_final\Gaussian filter 5x5\tb_gauss\gauss_Subsystem_find%5FkeyPoint_calculate%5Fkey%5Fpoint_line%5Fbuff%5F3x2_Delay10.fixedpointlog  use_init=on  reset_value=0
  Delay2 : allblocks_alteradspbuilder2/Delay  pipeline=1  pipeline_display=1  ClockPhase=1  use_ena=on  use_sclr=on  allowFloatingPointOverride=on  logOutputs=off  logFile=C:\Users\ASUS\Desktop\sift_fpga_final\Gaussian filter 5x5\tb_gauss\gauss_Subsystem_find%5FkeyPoint_calculate%5Fkey%5Fpoint_line%5Fbuff%5F3x2_Delay2.fixedpointlog  use_init=on  reset_value=0
  Delay5 : allblocks_alteradspbuilder2/Delay  pipeline=1  pipeline_display=1  ClockPhase=1  use_ena=on  use_sclr=on  allowFloatingPointOverride=on  logOutputs=off  logFile=C:\Users\ASUS\Desktop\sift_fpga_final\Gaussian filter 5x5\tb_gauss\gauss_Subsystem_find%5FkeyPoint_calculate%5Fkey%5Fpoint_line%5Fbuff%5F3x2_Delay5.fixedpointlog  use_init=on  reset_value=0
  Delay6 : allblocks_alteradspbuilder2/Delay  pipeline=1  pipeline_display=1  ClockPhase=1  use_ena=on  use_sclr=on  allowFloatingPointOverride=on  logOutputs=off  logFile=C:\Users\ASUS\Desktop\sift_fpga_final\Gaussian filter 5x5\tb_gauss\gauss_Subsystem_find%5FkeyPoint_calculate%5Fkey%5Fpoint_line%5Fbuff%5F3x2_Delay6.fixedpointlog  use_init=on  reset_value=0
  Delay9 : allblocks_alteradspbuilder2/Delay  pipeline=1  pipeline_display=1  ClockPhase=1  use_ena=on  use_sclr=on  allowFloatingPointOverride=on  logOutputs=off  logFile=C:\Users\ASUS\Desktop\sift_fpga_final\Gaussian filter 5x5\tb_gauss\gauss_Subsystem_find%5FkeyPoint_calculate%5Fkey%5Fpoint_line%5Fbuff%5F3x2_Delay9.fixedpointlog  use_init=on  reset_value=0
  Memory Delay : allblocks_alteradspbuilder2/Memory Delay  BusType=Unsigned Integer  bwl=8  bwr=0  pipeline=638  pipeline_display=638  ram_type=AUTO  use_ena=on  use_sclr=on  allowFloatingPointOverride=on  logOutputs=off  logFile=C:\Users\ASUS\Desktop\sift_fpga_final\Gaussian filter 5x5\tb_gauss\gauss_Subsystem_find%5FkeyPoint_calculate%5Fkey%5Fpoint_line%5Fbuff%5F3x2_Memory+Delay.fixedpointlog
  Memory Delay1 : allblocks_alteradspbuilder2/Memory Delay  BusType=Unsigned Integer  bwl=8  bwr=0  pipeline=638  pipeline_display=638  ram_type=AUTO  use_ena=on  use_sclr=on  allowFloatingPointOverride=on  logOutputs=off  logFile=C:\Users\ASUS\Desktop\sift_fpga_final\Gaussian filter 5x5\tb_gauss\gauss_Subsystem_find%5FkeyPoint_calculate%5Fkey%5Fpoint_line%5Fbuff%5F3x2_Memory+Delay1.fixedpointlog
  Out00 : Outport
  Out01 : Outport  Port=2
  Out02 : Outport  Port=3
  Out10 : Outport  Port=4
  Out11 : Outport  Port=5
  Out12 : Outport  Port=6
  Out20 : Outport  Port=7
  Out21 : Outport  Port=8
  Out22 : Outport  Port=9
  wires:
  Delay1/1 -> [data_01], Delay2/1
  Delay/1 -> [data_00], Delay1/1
  Delay9/1 -> [data_21], Delay10/1
  [clken] -> Delay10/2
  [clken] -> Memory Delay1/2
  Delay6/1 -> Memory Delay1/1, [data_12]
  Memory Delay1/1 -> [data_20], Delay9/1
  [clken] -> Delay9/2
  [data_02] -> Out02/1
  [clken] -> Delay1/2
  [clken] -> Delay/2
  [data_in] -> Delay/1
  [clken] -> Delay2/2
  Delay2/1 -> [data_02], Memory Delay/1
  [data_22] -> Out22/1
  Delay10/1 -> [data_22]
  clken/1 -> [clken]
  [data_21] -> Out21/1
  [data_20] -> Out20/1
  [data_10] -> Out10/1
  Memory Delay/1 -> [data_10], Delay5/1
  [clken] -> Memory Delay/2
  [clken] -> Delay6/2
  Delay5/1 -> [data_11], Delay6/1
  [data_12] -> Out12/1
  [data_00] -> Out00/1
  [data_01] -> Out01/1
  [clken] -> Delay5/2
  [data_11] -> Out11/1
  dataIn/1 -> [data_in]
  sclr/1 -> [sclr]
  [sclr] -> Delay/3
  [sclr] -> Delay1/3
  [sclr] -> Delay2/3
  [sclr] -> Memory Delay/3
  [sclr] -> Delay5/3
  [sclr] -> Delay6/3
  [sclr] -> Memory Delay1/3
  [sclr] -> Delay9/3
  [sclr] -> Delay10/3

== system showKeyPoint/Subsystem/find_keyPoint/calculate_key_point/line_buff_3x3 ==
  dataIn : Inport
  clken : Inport  Port=2
  sclr : Inport  Port=3
  Delay : allblocks_alteradspbuilder2/Delay  pipeline=1  pipeline_display=1  ClockPhase=1  use_ena=on  use_sclr=on  allowFloatingPointOverride=on  logOutputs=off  logFile=C:\Users\ASUS\Desktop\sift_fpga_final\Gaussian filter 5x5\tb_gauss\gauss_Subsystem_find%5FkeyPoint_calculate%5Fkey%5Fpoint_line%5Fbuff%5F3x3_Delay.fixedpointlog  use_init=on  reset_value=0
  Delay1 : allblocks_alteradspbuilder2/Delay  pipeline=1  pipeline_display=1  ClockPhase=1  use_ena=on  use_sclr=on  allowFloatingPointOverride=on  logOutputs=off  logFile=C:\Users\ASUS\Desktop\sift_fpga_final\Gaussian filter 5x5\tb_gauss\gauss_Subsystem_find%5FkeyPoint_calculate%5Fkey%5Fpoint_line%5Fbuff%5F3x3_Delay1.fixedpointlog  use_init=on  reset_value=0
  Delay10 : allblocks_alteradspbuilder2/Delay  pipeline=1  pipeline_display=1  ClockPhase=1  use_ena=on  use_sclr=on  allowFloatingPointOverride=on  logOutputs=off  logFile=C:\Users\ASUS\Desktop\sift_fpga_final\Gaussian filter 5x5\tb_gauss\gauss_Subsystem_find%5FkeyPoint_calculate%5Fkey%5Fpoint_line%5Fbuff%5F3x3_Delay10.fixedpointlog  use_init=on  reset_value=0
  Delay2 : allblocks_alteradspbuilder2/Delay  pipeline=1  pipeline_display=1  ClockPhase=1  use_ena=on  use_sclr=on  allowFloatingPointOverride=on  logOutputs=off  logFile=C:\Users\ASUS\Desktop\sift_fpga_final\Gaussian filter 5x5\tb_gauss\gauss_Subsystem_find%5FkeyPoint_calculate%5Fkey%5Fpoint_line%5Fbuff%5F3x3_Delay2.fixedpointlog  use_init=on  reset_value=0
  Delay5 : allblocks_alteradspbuilder2/Delay  pipeline=1  pipeline_display=1  ClockPhase=1  use_ena=on  use_sclr=on  allowFloatingPointOverride=on  logOutputs=off  logFile=C:\Users\ASUS\Desktop\sift_fpga_final\Gaussian filter 5x5\tb_gauss\gauss_Subsystem_find%5FkeyPoint_calculate%5Fkey%5Fpoint_line%5Fbuff%5F3x3_Delay5.fixedpointlog  use_init=on  reset_value=0
  Delay6 : allblocks_alteradspbuilder2/Delay  pipeline=1  pipeline_display=1  ClockPhase=1  use_ena=on  use_sclr=on  allowFloatingPointOverride=on  logOutputs=off  logFile=C:\Users\ASUS\Desktop\sift_fpga_final\Gaussian filter 5x5\tb_gauss\gauss_Subsystem_find%5FkeyPoint_calculate%5Fkey%5Fpoint_line%5Fbuff%5F3x3_Delay6.fixedpointlog  use_init=on  reset_value=0
  Delay9 : allblocks_alteradspbuilder2/Delay  pipeline=1  pipeline_display=1  ClockPhase=1  use_ena=on  use_sclr=on  allowFloatingPointOverride=on  logOutputs=off  logFile=C:\Users\ASUS\Desktop\sift_fpga_final\Gaussian filter 5x5\tb_gauss\gauss_Subsystem_find%5FkeyPoint_calculate%5Fkey%5Fpoint_line%5Fbuff%5F3x3_Delay9.fixedpointlog  use_init=on  reset_value=0
  Memory Delay : allblocks_alteradspbuilder2/Memory Delay  BusType=Unsigned Integer  bwl=8  bwr=0  pipeline=638  pipeline_display=638  ram_type=AUTO  use_ena=on  use_sclr=on  allowFloatingPointOverride=on  logOutputs=off  logFile=C:\Users\ASUS\Desktop\sift_fpga_final\Gaussian filter 5x5\tb_gauss\gauss_Subsystem_find%5FkeyPoint_calculate%5Fkey%5Fpoint_line%5Fbuff%5F3x3_Memory+Delay.fixedpointlog
  Memory Delay1 : allblocks_alteradspbuilder2/Memory Delay  BusType=Unsigned Integer  bwl=8  bwr=0  pipeline=638  pipeline_display=638  ram_type=AUTO  use_ena=on  use_sclr=on  allowFloatingPointOverride=on  logOutputs=off  logFile=C:\Users\ASUS\Desktop\sift_fpga_final\Gaussian filter 5x5\tb_gauss\gauss_Subsystem_find%5FkeyPoint_calculate%5Fkey%5Fpoint_line%5Fbuff%5F3x3_Memory+Delay1.fixedpointlog
  Out00 : Outport
  Out01 : Outport  Port=2
  Out02 : Outport  Port=3
  Out10 : Outport  Port=4
  Out11 : Outport  Port=5
  Out12 : Outport  Port=6
  Out20 : Outport  Port=7
  Out21 : Outport  Port=8
  Out22 : Outport  Port=9
  wires:
  Delay1/1 -> [data_01], Delay2/1
  Delay/1 -> [data_00], Delay1/1
  Delay9/1 -> [data_21], Delay10/1
  [clken] -> Delay10/2
  [clken] -> Memory Delay1/2
  Delay6/1 -> Memory Delay1/1, [data_12]
  Memory Delay1/1 -> [data_20], Delay9/1
  [clken] -> Delay9/2
  [data_02] -> Out02/1
  [clken] -> Delay1/2
  [clken] -> Delay/2
  [data_in] -> Delay/1
  [clken] -> Delay2/2
  Delay2/1 -> [data_02], Memory Delay/1
  [data_22] -> Out22/1
  Delay10/1 -> [data_22]
  clken/1 -> [clken]
  [data_21] -> Out21/1
  [data_20] -> Out20/1
  [data_10] -> Out10/1
  Memory Delay/1 -> [data_10], Delay5/1
  [clken] -> Memory Delay/2
  [clken] -> Delay6/2
  Delay5/1 -> [data_11], Delay6/1
  [data_12] -> Out12/1
  [data_00] -> Out00/1
  [data_01] -> Out01/1
  [clken] -> Delay5/2
  [data_11] -> Out11/1
  dataIn/1 -> [data_in]
  sclr/1 -> [sclr]
  [sclr] -> Delay/3
  [sclr] -> Delay1/3
  [sclr] -> Delay2/3
  [sclr] -> Memory Delay/3
  [sclr] -> Delay5/3
  [sclr] -> Delay6/3
  [sclr] -> Memory Delay1/3
  [sclr] -> Delay9/3
  [sclr] -> Delay10/3

== system showKeyPoint/Subsystem/find_keyPoint/scale_space/Gaussian_scale1 ==
  pixel_in : Inport
  valid_in : Inport  Port=2
  sclr : Inport  Port=3
  Mul : Subsystem
  Round : allblocks_alteradspbuilder2/Round  BusType=Signed Fractional  bwl=9  bwr=16  bitsToRemove=0  roundMode=TRUNCATE_LOW  userRoundMode=Truncate  pipeline=off  pipeline_display=0  use_ena=off  use_aclr=off
  line_buff : Subsystem
  pixel_out : Outport
  wires:
  Mul/1(pixel) -> Round/1
  Round/1 -> pixel_out/1
  line_buff/20(Out34) -> Mul/20(In34)
  line_buff/7(Out11) -> Mul/7(In11)
  line_buff/22(Out41) -> Mul/22(In41)
  line_buff/21(Out40) -> Mul/21(In40)
  line_buff/23(Out42) -> Mul/23(In42)
  line_buff/24(Out43) -> Mul/24(In43)
  line_buff/6(Out10) -> Mul/6(In10)
  line_buff/19(Out33) -> Mul/19(In33)
  line_buff/25(Out44) -> Mul/25(In44)
  line_buff/11(Out20) -> Mul/11(In20)
  line_buff/1(Out00) -> Mul/1(In00)
  line_buff/5(Out04) -> Mul/5(In04)
  pixel_in/1 -> line_buff/1(dataIn)
  line_buff/13(Out22) -> Mul/13(In22)
  line_buff/16(Out30) -> Mul/16(In30)
  line_buff/18(Out32) -> Mul/18(In32)
  line_buff/10(Out14) -> Mul/10(In14)
  valid_in/1 -> Mul/26(clken), line_buff/2(clken)
  line_buff/12(Out21) -> Mul/12(In21)
  line_buff/14(Out23) -> Mul/14(In23)
  line_buff/2(Out01) -> Mul/2(In01)
  line_buff/4(Out03) -> Mul/4(In03)
  line_buff/9(Out13) -> Mul/9(In13)
  line_buff/15(Out24) -> Mul/15(In24)
  line_buff/17(Out31) -> Mul/17(In31)
  line_buff/3(Out02) -> Mul/3(In02)
  line_buff/8(Out12) -> Mul/8(In12)
  sclr/1 -> Mul/27(sclr), line_buff/3(sclr)

== system showKeyPoint/Subsystem/find_keyPoint/scale_space/Gaussian_scale2 ==
  pixel_in : Inport
  valid_in : Inport  Port=2
  sclr : Inport  Port=3
  Mul : Subsystem
  Round : allblocks_alteradspbuilder2/Round  BusType=Signed Fractional  bwl=9  bwr=16  bitsToRemove=0  roundMode=TRUNCATE_LOW  userRoundMode=Truncate  pipeline=off  pipeline_display=0  use_ena=off  use_aclr=off
  line_buff : Subsystem
  pixel_out : Outport
  wires:
  Mul/1(pixel) -> Round/1
  Round/1 -> pixel_out/1
  line_buff/20(Out34) -> Mul/20(In34)
  line_buff/7(Out11) -> Mul/7(In11)
  line_buff/22(Out41) -> Mul/22(In41)
  line_buff/21(Out40) -> Mul/21(In40)
  line_buff/23(Out42) -> Mul/23(In42)
  line_buff/24(Out43) -> Mul/24(In43)
  line_buff/6(Out10) -> Mul/6(In10)
  line_buff/19(Out33) -> Mul/19(In33)
  line_buff/25(Out44) -> Mul/25(In44)
  line_buff/11(Out20) -> Mul/11(In20)
  line_buff/1(Out00) -> Mul/1(In00)
  line_buff/5(Out04) -> Mul/5(In04)
  pixel_in/1 -> line_buff/1(dataIn)
  line_buff/13(Out22) -> Mul/13(In22)
  line_buff/16(Out30) -> Mul/16(In30)
  line_buff/18(Out32) -> Mul/18(In32)
  line_buff/10(Out14) -> Mul/10(In14)
  valid_in/1 -> Mul/26(clken), line_buff/2(clken)
  line_buff/12(Out21) -> Mul/12(In21)
  line_buff/14(Out23) -> Mul/14(In23)
  line_buff/2(Out01) -> Mul/2(In01)
  line_buff/4(Out03) -> Mul/4(In03)
  line_buff/9(Out13) -> Mul/9(In13)
  line_buff/15(Out24) -> Mul/15(In24)
  line_buff/17(Out31) -> Mul/17(In31)
  line_buff/3(Out02) -> Mul/3(In02)
  line_buff/8(Out12) -> Mul/8(In12)
  sclr/1 -> Mul/27(sclr), line_buff/3(sclr)

== system showKeyPoint/Subsystem/find_keyPoint/scale_space/Gaussian_scale3 ==
  pixel_in : Inport
  valid_in : Inport  Port=2
  sclr : Inport  Port=3
  Mul : Subsystem
  Round : allblocks_alteradspbuilder2/Round  BusType=Signed Fractional  bwl=9  bwr=16  bitsToRemove=0  roundMode=TRUNCATE_LOW  userRoundMode=Truncate  pipeline=off  pipeline_display=0  use_ena=off  use_aclr=off
  line_buff : Subsystem
  pixel_out : Outport
  wires:
  Mul/1(pixel) -> Round/1
  Round/1 -> pixel_out/1
  line_buff/20(Out34) -> Mul/20(In34)
  line_buff/7(Out11) -> Mul/7(In11)
  line_buff/22(Out41) -> Mul/22(In41)
  line_buff/21(Out40) -> Mul/21(In40)
  line_buff/23(Out42) -> Mul/23(In42)
  line_buff/24(Out43) -> Mul/24(In43)
  line_buff/6(Out10) -> Mul/6(In10)
  line_buff/19(Out33) -> Mul/19(In33)
  line_buff/25(Out44) -> Mul/25(In44)
  line_buff/11(Out20) -> Mul/11(In20)
  line_buff/1(Out00) -> Mul/1(In00)
  line_buff/5(Out04) -> Mul/5(In04)
  pixel_in/1 -> line_buff/1(dataIn)
  line_buff/13(Out22) -> Mul/13(In22)
  line_buff/16(Out30) -> Mul/16(In30)
  line_buff/18(Out32) -> Mul/18(In32)
  line_buff/10(Out14) -> Mul/10(In14)
  valid_in/1 -> Mul/26(clken), line_buff/2(clken)
  line_buff/12(Out21) -> Mul/12(In21)
  line_buff/14(Out23) -> Mul/14(In23)
  line_buff/2(Out01) -> Mul/2(In01)
  line_buff/4(Out03) -> Mul/4(In03)
  line_buff/9(Out13) -> Mul/9(In13)
  line_buff/15(Out24) -> Mul/15(In24)
  line_buff/17(Out31) -> Mul/17(In31)
  line_buff/3(Out02) -> Mul/3(In02)
  line_buff/8(Out12) -> Mul/8(In12)
  sclr/1 -> Mul/27(sclr), line_buff/3(sclr)

== system showKeyPoint/Subsystem/find_keyPoint/scale_space/Gaussian_scale4 ==
  pixel_in : Inport
  valid_in : Inport  Port=2
  sclr : Inport  Port=3
  Mul : Subsystem
  Round : allblocks_alteradspbuilder2/Round  BusType=Signed Fractional  bwl=9  bwr=16  bitsToRemove=0  roundMode=TRUNCATE_LOW  userRoundMode=Truncate  pipeline=off  pipeline_display=0  use_ena=off  use_aclr=off
  line_buff : Subsystem
  pixel_out : Outport
  wires:
  line_buff/20(Out34) -> Mul/20(In34)
  line_buff/7(Out11) -> Mul/7(In11)
  line_buff/22(Out41) -> Mul/22(In41)
  line_buff/21(Out40) -> Mul/21(In40)
  line_buff/23(Out42) -> Mul/23(In42)
  line_buff/24(Out43) -> Mul/24(In43)
  line_buff/6(Out10) -> Mul/6(In10)
  line_buff/19(Out33) -> Mul/19(In33)
  line_buff/25(Out44) -> Mul/25(In44)
  line_buff/11(Out20) -> Mul/11(In20)
  line_buff/1(Out00) -> Mul/1(In00)
  line_buff/5(Out04) -> Mul/5(In04)
  pixel_in/1 -> line_buff/1(dataIn)
  line_buff/13(Out22) -> Mul/13(In22)
  line_buff/16(Out30) -> Mul/16(In30)
  line_buff/18(Out32) -> Mul/18(In32)
  Mul/1(pixel) -> Round/1
  line_buff/10(Out14) -> Mul/10(In14)
  valid_in/1 -> Mul/26(clken), line_buff/2(clken)
  line_buff/12(Out21) -> Mul/12(In21)
  line_buff/14(Out23) -> Mul/14(In23)
  line_buff/2(Out01) -> Mul/2(In01)
  line_buff/4(Out03) -> Mul/4(In03)
  line_buff/9(Out13) -> Mul/9(In13)
  line_buff/15(Out24) -> Mul/15(In24)
  line_buff/17(Out31) -> Mul/17(In31)
  line_buff/3(Out02) -> Mul/3(In02)
  line_buff/8(Out12) -> Mul/8(In12)
  Round/1 -> pixel_out/1
  sclr/1 -> Mul/27(sclr), line_buff/3(sclr)
